simulink subsystem "Plant_Attitude"  (R2025a)
settings: Solver=VariableStepAuto  StartTime=0.0  StopTime=10.0  RelTol=1e-3
undefined symbols (not defined in the file): J, Jinv, q0, w0
libraries: matrix_library x1
settings Model: Creator=Jackt  LastModifiedBy=Jackt

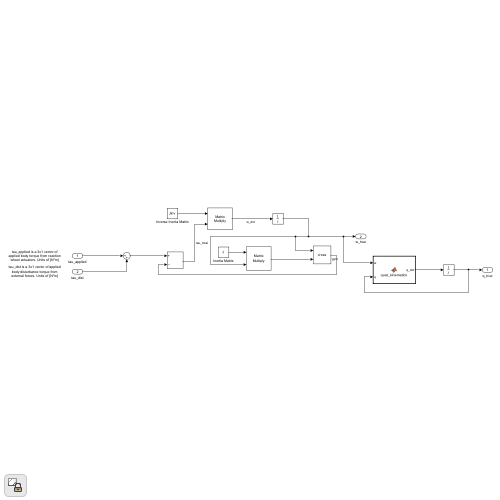
[thumbnail: Simulink's stored preview of the top-level diagram]
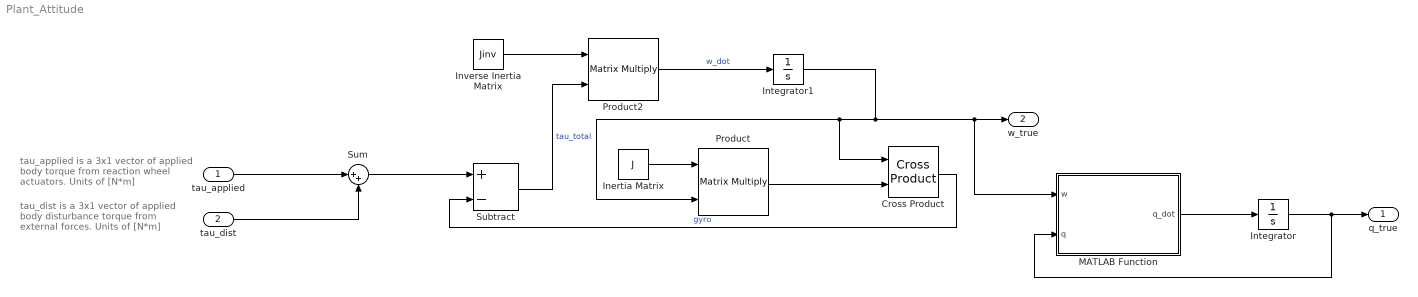
== system Plant_Attitude ==
  note: tau_applied is a 3x1 vector of applied body torque from reaction wheel actuators. Units of [N*m]
  note: tau_dist is a 3x1 vector of applied body disturbance torque from external forces. Units of [N*m]
  tau_applied : Inport  Unit=N*m
  tau_dist : Inport  Port=2  Unit=N*m
  Cross Product : matrix_library/Cross Product
  Inertia Matrix : Constant  Value=J
  Integrator : Integrator  InitialCondition=q0
  Integrator1 : Integrator  InitialCondition=w0
  Inverse Inertia Matrix : Constant  Value=Jinv
  MATLAB Function : MATLAB Function  TreatAsAtomicUnit=on
  Product : Product  Multiplication=Matrix(*)
  Product2 : Product  Multiplication=Matrix(*)
  Subtract : Sum  Inputs=+-
  Sum : Sum  Inputs=|++
  q_true : Outport
  w_true : Outport  Port=2
  wires:
  Inertia Matrix/1 -> Product/1
  Subtract/1 -> Product2/2  "tau_total"
  Sum/1 -> Subtract/1
  tau_applied/1 -> Sum/1
  Inverse Inertia Matrix/1 -> Product2/1
  tau_dist/1 -> Sum/2
  Product2/1 -> Integrator1/1  "w_dot"
  Integrator1/1 -> w_true/1, MATLAB Function/1(w), Product/2, Cross Product/1
  Cross Product/1 -> Subtract/2  "gyro"
  MATLAB Function/1(q_dot) -> Integrator/1
  Product/1 -> Cross Product/2
  Integrator/1 -> q_true/1, MATLAB Function/2(q)

== matlab function Plant_Attitude/MATLAB Function ==
  data: w input; q_dot output size=[4 1]; q input
function q_dot = quat_kinematics(w, q)
% q is scalar-first [q0;q1;q2;q3], w = [wx;wy;wz]
wx = w(1); wy = w(2); wz = w(3);

Omega = [ 0   -wx  -wy  -wz;
          wx   0    wz  -wy;
          wy  -wz   0    wx;
          wz   wy  -wx   0 ];

q_dot = 0.5 * Omega * q;
end
